simulink library "Murphy_SimscapeElectrical"  (R2019a)
settings: Solver=VariableStepAuto  StartTime=0.0  StopTime=10.0  RelTol=1e-3
libraries: fl_lib x8, nesl_utility x5
settings Model: Creator=Matt  LastModifiedBy=Matt

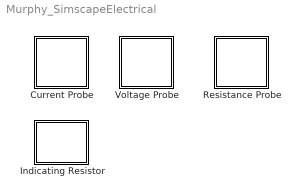
== system Murphy_SimscapeElectrical ==
  "Current Probe " : Subsystem  BlockKeywords=__PRM__SERIALIZED__DATA__:Current Probe,Ammeter  mask{ShowInLibBrowser=on}
      mask init:
      | set_param(gcb, 'BlockKeywords', {'Current Probe', 'Ammeter'});
      settings: OpenFcn=open_system(gcb,'Mask');
      mask Display:
      | disp('A');
      | port_label('lconn', 1, '+');
      | port_label('rconn', 1, '-');
  Indicating Resistor : Subsystem  BlockKeywords=__PRM__SERIALIZED__DATA__:Indicating Resistor  mask{ShowInLibBrowser=on, amps=0, volts=0, resistance=10}
      mask init:
      | set_param(gcb, 'BlockKeywords', {'Indicating Resistor'});
      settings: OpenFcn=open_system(gcb,'Mask');
      mask Display:
      | orient = get_param(gcb, 'Orientation');
      | pos = get_param(gcb, 'Position');
      | 
      | width = pos(3) - pos(1);
      | height = pos(4) - pos(2);
      | 
      | if startsWith(orient, 'up') || startsWith(orient, 'down')
      |     ww = width; width = height; height = ww;
      | end
      | 
      | sawTeeth = [0 1 -1 1 -1 1 -1 1 -1 0];
      | 
      | sawWidthGap = width - 20;
      | if (sawWidthGap < 20) sawWidthGap = width*0.5; end
      | sawWidthRatio = sawWidthGap / width;
      | sawWidth = max(1,(width*sawWidthRatio) - mod(width*sawWidthRatio, length(sawTeeth)));
      | sawStep = sawWidth / length(sawTeeth);
      | sawXs = 0:sawStep:(length(sawTeeth)-1)*sawStep;
      | 
      | sawCentered = width / 2 - (sawWidth-sawStep) / 2;
      | sawStart = sawCentered;%marginLeft/2 + + sawStep/4 + floor(width / 2 - sawWidth / 2);
      | 
      | marginLeft = 15;
      | if (sawStart < marginLeft), marginLeft = sawStart; end;
      | marginRight = width - marginLeft;
      | 
      | sawXs(1) = sawStep/2;
      | sawXs(end) = sawXs(end) - sawStep/2;
      | 
      | xs = [marginLeft sawStart+sawXs marginRight];
      | 
      | ys = [0.5 0.5 + 0.1*[sawTeeth] 0.5];
      | ys = height - ys*height;
      | 
      | if startsWith(orient, 'up') || startsWith(orient, 'down')
      |     xxs = xs; xs = ys; ys = xxs;
      | end
      | 
      | plot(xs, ys);
      | 
      | port_label('lconn', 1, '+');
      | port_label('rconn', 1, '-');
      | 
      | amps = [get_param(gcb, 'amps') ' A'];
      | volts = [get_param(gcb, 'volts') ' V'];
      | 
      | if startsWith(orient, 'up') || startsWith(orient, 'down')
      |   text(height, width/2, amps, 'horizontalAlignment', 'right', 'verticalAlignment', 'middle')
      |   text(0, width/2, volts, 'horizontalAlignment', 'left', 'verticalAlignment', 'middle')
      | else
      |   text(width/2, height, volts, 'horizontalAlignment', 'center', 'verticalAlignment', 'top')
      |   text(width/2, 0, amps, 'horizontalAlignment', 'center', 'verticalAlignment', 'bottom')
      | end
  Resistance Probe : Subsystem  BlockKeywords=__PRM__SERIALIZED__DATA__:Resistance Probe,ohmmeter  mask{ShowInLibBrowser=on}
      mask init:
      | set_param(gcb, 'BlockKeywords', {'Resistance Probe', 'ohmmeter'});
      settings: OpenFcn=open_system(gcb,'Mask');
      mask Display:
      | disp('Ω');
      | port_label('lconn', 1, '+');
      | port_label('rconn', 1, '-');
  Voltage Probe : Subsystem  BlockKeywords=__PRM__SERIALIZED__DATA__:Voltage Probe,voltmeter  mask{ShowInLibBrowser=on}
      mask init:
      | set_param(gcb, 'BlockKeywords', {'Voltage Probe', 'voltmeter'});
      settings: OpenFcn=open_system(gcb,'Mask');
      mask Display:
      | disp('V');
      | port_label('lconn', 1, '+');
      | port_label('rconn', 1, '-');

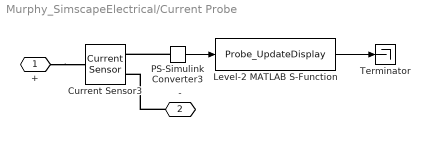
== system Murphy_SimscapeElectrical/Current Probe  ==
  Current Sensor3 : fl_lib/Electrical/Electrical Sensors/Current Sensor
  Level-2 MATLAB S-Function : M-S-Function  FunctionName=Probe_UpdateDisplay  Parameters='A'
  PS-Simulink Converter3 : nesl_utility/PS-Simulink Converter  PhysicalDomain=network_engine_domain  SubClassName=ps_output  LeftPortType=input  RightPortType=output  PseudoPeriodic=off  Frequencies=[]  Unit=A  AffineConversion=off
  Terminator : Terminator
  + : PMIOPort  Side=Left
  - : PMIOPort  Port=2  Side=Right
  wires:
  PS-Simulink Converter3/1 -> Level-2 MATLAB S-Function/1
  Level-2 MATLAB S-Function/1 -> Terminator/1
  connections:
  PS-Simulink Converter3/LConn1 -- Current Sensor3/RConn1
  -/RConn1 -- Current Sensor3/RConn2
  +/RConn1 -- Current Sensor3/LConn1

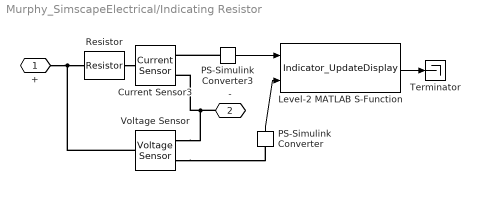
== system Murphy_SimscapeElectrical/Indicating Resistor ==
  Current Sensor3 : fl_lib/Electrical/Electrical Sensors/Current Sensor
  Level-2 MATLAB S-Function : M-S-Function  FunctionName=Indicator_UpdateDisplay
  PS-Simulink Converter : nesl_utility/PS-Simulink Converter  PhysicalDomain=network_engine_domain  SubClassName=ps_output  LeftPortType=input  RightPortType=output  PseudoPeriodic=off  Frequencies=[]  Unit=1  AffineConversion=off
  PS-Simulink Converter3 : nesl_utility/PS-Simulink Converter  PhysicalDomain=network_engine_domain  SubClassName=ps_output  LeftPortType=input  RightPortType=output  PseudoPeriodic=off  Frequencies=[]  Unit=A  AffineConversion=off
  Resistor : fl_lib/Electrical/Electrical Elements/Resistor  R=resistance Ohm  i_specify=off  i_priority=None  i=0 A  i_nominal_specify=off  i_nominal_unit=A  i_nominal_value=1  v_specify=off  v_priority=None  v=0 V  v_nominal_specify=off  v_nominal_unit=V  v_nominal_value=1
  Terminator : Terminator
  Voltage Sensor : fl_lib/Electrical/Electrical Sensors/Voltage Sensor
  + : PMIOPort  Side=Left
  - : PMIOPort  Port=2  Side=Right
  wires:
  Level-2 MATLAB S-Function/1 -> Terminator/1
  PS-Simulink Converter3/1 -> Level-2 MATLAB S-Function/1
  PS-Simulink Converter/1 -> Level-2 MATLAB S-Function/2
  connections:
  +/RConn1 -- Voltage Sensor/LConn1 -- Resistor/LConn1
  -/RConn1 -- Voltage Sensor/RConn2 -- Current Sensor3/RConn2
  PS-Simulink Converter3/LConn1 -- Current Sensor3/RConn1
  Voltage Sensor/RConn1 -- PS-Simulink Converter/LConn1
  Resistor/RConn1 -- Current Sensor3/LConn1

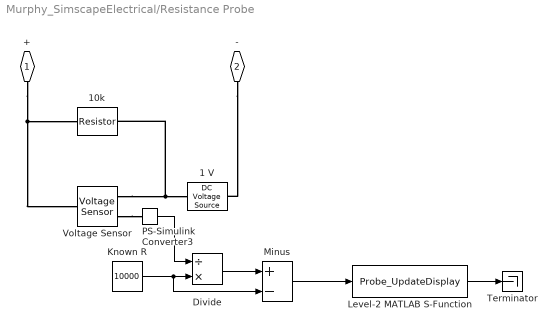
== system Murphy_SimscapeElectrical/Resistance Probe ==
  1 V : fl_lib/Electrical/Electrical Sources/DC Voltage Source  v0=1 V
  10k : fl_lib/Electrical/Electrical Elements/Resistor  R=10 kOhm  i_specify=off  i_priority=None  i=0 A  i_nominal_specify=off  i_nominal_unit=A  i_nominal_value=1  v_specify=off  v_priority=None  v=0 V  v_nominal_specify=off  v_nominal_unit=V  v_nominal_value=1
  Divide : Product  Inputs=/*
  Known R : Constant  Value=10000
  Level-2 MATLAB S-Function : M-S-Function  FunctionName=Probe_UpdateDisplay  Parameters=suffix  mask{suffix='ohm'}
      mask prompts: suffix "Unit Suffix"
  Minus : Sum  Inputs=+-
  PS-Simulink Converter3 : nesl_utility/PS-Simulink Converter  PhysicalDomain=network_engine_domain  SubClassName=ps_output  LeftPortType=input  RightPortType=output  PseudoPeriodic=off  Frequencies=[]  Unit=1  AffineConversion=off
  Terminator : Terminator
  Voltage Sensor : fl_lib/Electrical/Electrical Sensors/Voltage Sensor
  + : PMIOPort  Side=Left
  - : PMIOPort  Port=2  Side=Right
  wires:
  Level-2 MATLAB S-Function/1 -> Terminator/1
  PS-Simulink Converter3/1 -> Divide/1
  Divide/1 -> Minus/1
  Known R/1 -> Minus/2, Divide/2
  Minus/1 -> Level-2 MATLAB S-Function/1
  connections:
  +/RConn1 -- Voltage Sensor/LConn1 -- 10k/LConn1
  Voltage Sensor/RConn2 -- 10k/RConn1 -- 1 V/RConn1
  Voltage Sensor/RConn1 -- PS-Simulink Converter3/LConn1
  -/RConn1 -- 1 V/LConn1

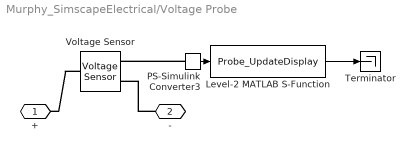
== system Murphy_SimscapeElectrical/Voltage Probe ==
  Level-2 MATLAB S-Function : M-S-Function  FunctionName=Probe_UpdateDisplay  Parameters=suffix  mask{suffix='V'}
      mask prompts: suffix "Unit Suffix"
  PS-Simulink Converter3 : nesl_utility/PS-Simulink Converter  PhysicalDomain=network_engine_domain  SubClassName=ps_output  LeftPortType=input  RightPortType=output  PseudoPeriodic=off  Frequencies=[]  Unit=V  AffineConversion=off
  Terminator : Terminator
  Voltage Sensor : fl_lib/Electrical/Electrical Sensors/Voltage Sensor
  + : PMIOPort  Side=Left
  - : PMIOPort  Port=2  Side=Right
  wires:
  Level-2 MATLAB S-Function/1 -> Terminator/1
  PS-Simulink Converter3/1 -> Level-2 MATLAB S-Function/1
  connections:
  Voltage Sensor/LConn1 -- +/RConn1
  -/RConn1 -- Voltage Sensor/RConn2
  PS-Simulink Converter3/LConn1 -- Voltage Sensor/RConn1
